simulink model "pendulum_v30"  (R2020b)
settings: Solver=FixedStepAuto  StartTime=0.0  StopTime=5  FixedStep=0.01  RelTol=1e-3
model workspace (MAT data in the model file):
  I = 0
  c = 0
  g = 9.81
  l = 1
  m = 1
  max_tau = 2
  theta0 = 0
  theta_dot0 = 0
settings Model: Creator=GWSZ  LastModifiedBy=mjj26
settings DataIOCC: SaveFormat=StructureWithTime
settings DebuggingCC: SFMachineParentedDataDiag=error

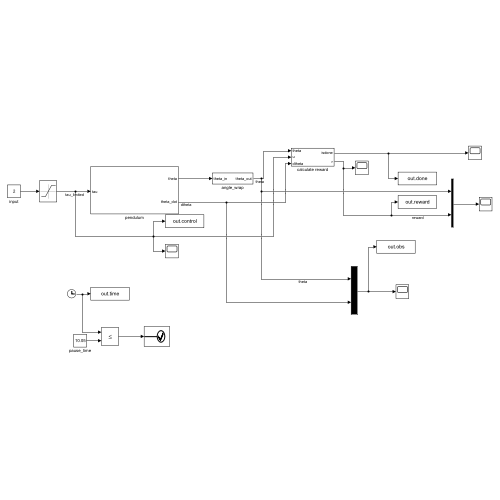
[thumbnail: Simulink's stored preview of the top-level diagram]
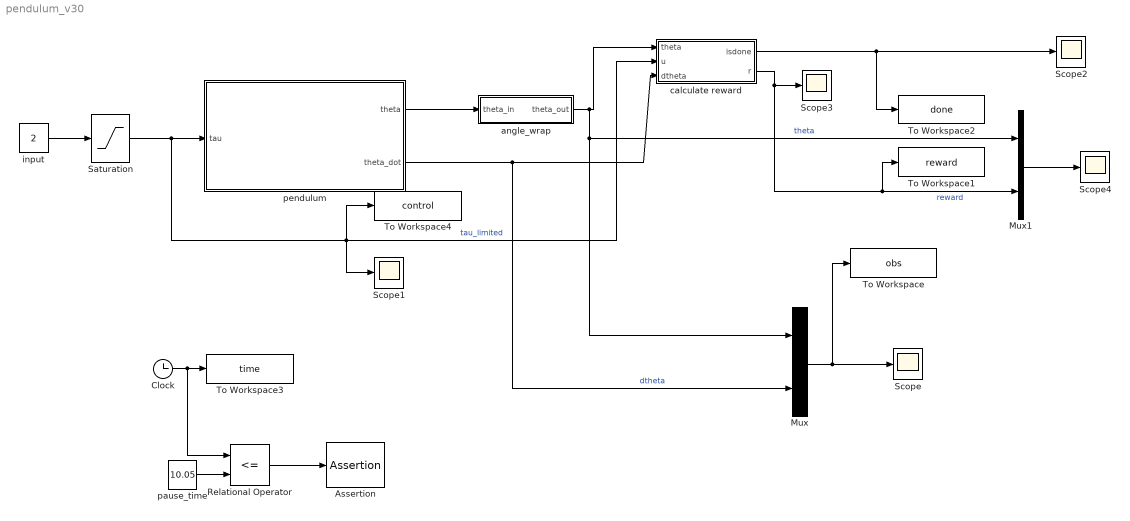
== system pendulum_v30 ==
  Assertion : Assertion  AssertionFailFcn=set_param(bdroot, 'SimulationCommand', 'pause');  StopWhenAssertionFail=off
  Clock : Clock
  Mux : Mux  Inputs=2
  Mux1 : Mux  Inputs=2
  Relational Operator : RelationalOperator  Operator=<=  OutDataTypeStr=boolean  RndMeth=Simplest
  Saturation : Saturate  UpperLimit=max_tau  LowerLimit=-max_tau
  Scope{,1..4} (5 alike) : Scope
  To Workspace : ToWorkspace  VariableName=obs  SaveFormat=Timeseries  SampleTime=-1
  To Workspace1 : ToWorkspace  VariableName=reward  SaveFormat=Timeseries  SampleTime=-1
  To Workspace2 : ToWorkspace  VariableName=done  SaveFormat=Timeseries  SampleTime=-1
  To Workspace3 : ToWorkspace  VariableName=time  SaveFormat=Timeseries  SampleTime=-1
  To Workspace4 : ToWorkspace  VariableName=control  SaveFormat=Timeseries  SampleTime=-1
  angle_wrap : Subsystem
  calculate reward : Subsystem
  input : Constant  Value=2
  pause_time : Constant  Value=10.05
  pendulum : Subsystem
  wires:
  input/1 -> Saturation/1
  Saturation/1 -> To Workspace4/1, Scope1/1, calculate reward/2(u), pendulum/1(tau)  "tau_limited"
  pendulum/1(theta) -> angle_wrap/1(theta_in)
  pendulum/2(theta_dot) -> Mux/2, calculate reward/3(dtheta)  "dtheta"
  angle_wrap/1(theta_out) -> calculate reward/1(theta), Mux/1, Mux1/1  "theta"
  Mux/1 -> To Workspace/1, Scope/1
  calculate reward/1(isdone) -> Scope2/1, To Workspace2/1
  calculate reward/2(r) -> To Workspace1/1, Mux1/2, Scope3/1  "reward"
  Mux1/1 -> Scope4/1
  Relational Operator/1 -> Assertion/1
  Clock/1 -> Relational Operator/1, To Workspace3/1
  pause_time/1 -> Relational Operator/2

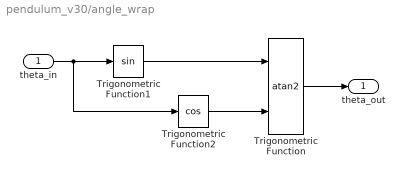
== system pendulum_v30/angle_wrap ==
  theta_in : Inport
  Trigonometric Function : Trigonometry  Operator=atan2
  Trigonometric Function1 : Trigonometry
  Trigonometric Function2 : Trigonometry  Operator=cos
  theta_out : Outport  VectorParamsAs1DForOutWhenUnconnected=off
  wires:
  theta_in/1 -> Trigonometric Function2/1, Trigonometric Function1/1
  Trigonometric Function/1 -> theta_out/1
  Trigonometric Function1/1 -> Trigonometric Function/1
  Trigonometric Function2/1 -> Trigonometric Function/2

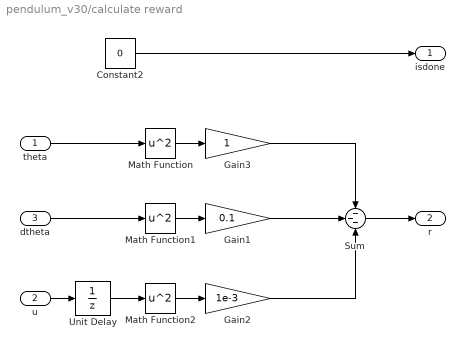
== system pendulum_v30/calculate reward ==
  theta : Inport
  u : Inport  Port=2
  dtheta : Inport  Port=3
  Constant2 : Constant  Value=0
  Gain1 : Gain  Gain=0.1
  Gain2 : Gain  Gain=1e-3
  Gain3 : Gain
  Math Function : Math  Operator=square  SignedPower=on  SaturateOnIntegerOverflow=on
  Math Function1 : Math  Operator=square  SignedPower=on  SaturateOnIntegerOverflow=on
  Math Function2 : Math  Operator=square  SignedPower=on  SaturateOnIntegerOverflow=on
  Sum : Sum  Inputs=---
  Unit Delay : UnitDelay  SampleTime=-1  HasFrameUpgradeWarning=on
  isdone : Outport  VectorParamsAs1DForOutWhenUnconnected=off
  r : Outport  Port=2  VectorParamsAs1DForOutWhenUnconnected=off
  wires:
  Constant2/1 -> isdone/1
  theta/1 -> Math Function/1
  dtheta/1 -> Math Function1/1
  u/1 -> Unit Delay/1
  Sum/1 -> r/1
  Math Function/1 -> Gain3/1
  Math Function1/1 -> Gain1/1
  Math Function2/1 -> Gain2/1
  Gain2/1 -> Sum/3
  Gain1/1 -> Sum/2
  Gain3/1 -> Sum/1
  Unit Delay/1 -> Math Function2/1

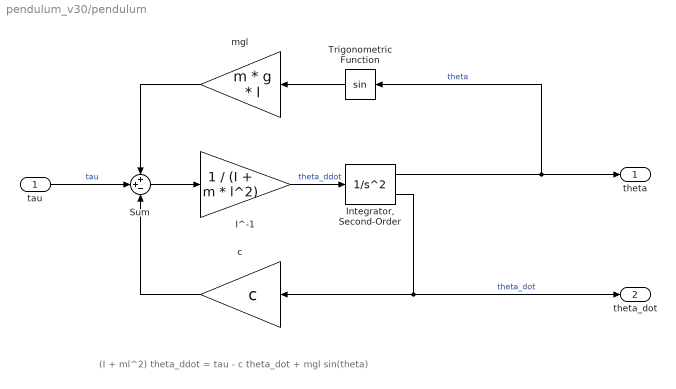
== system pendulum_v30/pendulum ==
  note: (I + ml^2) theta_ddot = tau - c theta_dot + mgl sin(theta)
  tau : Inport
  I^-1 : Gain  Gain=1 / (I + m * l^2)
  "Integrator, Second-Order" : SecondOrderIntegrator  ICX=theta0  UpperLimitX=1  LowerLimitX=0  StateNameX='theta'  ICDXDT=theta_dot0  StateNameDXDT='theta_dot'
  Sum : Sum  Inputs=++-
  Trigonometric Function : Trigonometry
  c : Gain  Gain=c
  mgl : Gain  Gain=m * g * l
  theta : Outport  VectorParamsAs1DForOutWhenUnconnected=off
  theta_dot : Outport  Port=2  VectorParamsAs1DForOutWhenUnconnected=off
  wires:
  mgl/1 -> Sum/1
  c/1 -> Sum/3
  Trigonometric Function/1 -> mgl/1
  Sum/1 -> I^-1/1
  "Integrator, Second-Order"/1 -> theta/1, Trigonometric Function/1  "theta"
  I^-1/1 -> "Integrator, Second-Order"/1  "theta_ddot"
  "Integrator, Second-Order"/2 -> c/1, theta_dot/1  "theta_dot"
  tau/1 -> Sum/2  "tau"
